simulink model "ai_neuron"  (R2020a)
settings: Solver=VariableStepAuto  StartTime=0.0  StopTime=30  RelTol=1e-3
libraries: xbsIndex_r4 x56, simulink x1
settings Model: Creator=Bunny1719  LastModifiedBy=asus

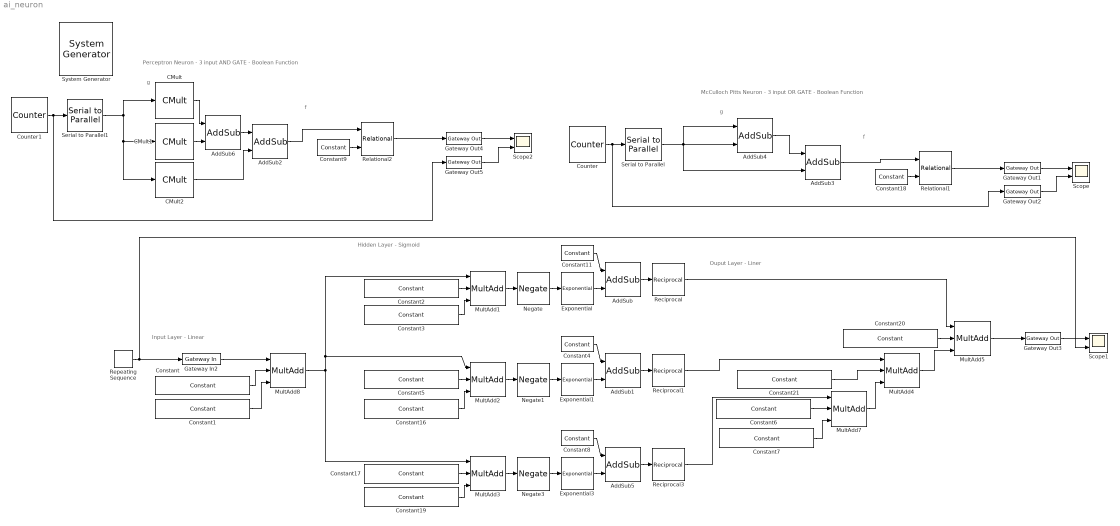
== system ai_neuron ==
  note: Ouput Layer - Liner
  note: Hidden Layer - Sigmoid
  note: Input Layer - Linear
  note: McCulloch Pitts Neuron - 3 input OR GATE - Boolean Function
  note: f
  note: g
  note: Perceptron Neuron - 3 input AND GATE - Boolean Function
  note: g
  note: f
  " System Generator" : xbsIndex_r4/ System Generator  Tag=genX  xilinxfamily=kintex7  part=xc7k325t  speed=-3  package=fbg676  synthesis_tool=Vivado  clock_wrapper=Clock Enables  directory=./netlist  proj_type=Vivado  Synth_file=Vivado Synthesis Defaults  Impl_file=Vivado Implementation Defaults  testbench=off  simulink_period=1  sysclk_period=10  dcm_input_clock_period=10  incr_netlist=off  trim_vbits=Everywhere in SubSystem  dbl_ovrd=According to Block Masks  core_generation=According to Block Masks  run_coregen=off  deprecated_control=off  eval_field=0  block_type=sysgen
  AddSub : xbsIndex_r4/AddSub  mode=Addition  use_carryin=off  use_carryout=off  en=off  latency=1  precision=Full  arith_type=Unsigned  n_bits=16  bin_pt=14  quantization=Truncate  overflow=Wrap  use_behavioral_HDL=off  hw_selection=Fabric  pipelined=off  dbl_ovrd=off  block_type=addsub
  AddSub1 : xbsIndex_r4/AddSub  mode=Addition  use_carryin=off  use_carryout=off  en=off  latency=1  precision=Full  arith_type=Unsigned  n_bits=16  bin_pt=14  quantization=Truncate  overflow=Wrap  use_behavioral_HDL=off  hw_selection=Fabric  pipelined=off  dbl_ovrd=off  block_type=addsub
  AddSub2 : xbsIndex_r4/AddSub  mode=Addition  use_carryin=off  use_carryout=off  en=off  latency=1  precision=User Defined  arith_type=Unsigned  n_bits=5  bin_pt=0  quantization=Truncate  overflow=Wrap  use_behavioral_HDL=off  hw_selection=Fabric  pipelined=off  dbl_ovrd=off  block_type=addsub
  AddSub3 : xbsIndex_r4/AddSub  mode=Addition  use_carryin=off  use_carryout=off  en=off  latency=1  precision=User Defined  arith_type=Unsigned  n_bits=3  bin_pt=0  quantization=Truncate  overflow=Wrap  use_behavioral_HDL=off  hw_selection=Fabric  pipelined=off  dbl_ovrd=off  block_type=addsub
  AddSub4 : xbsIndex_r4/AddSub  mode=Addition  use_carryin=off  use_carryout=off  en=off  latency=1  precision=User Defined  arith_type=Unsigned  n_bits=3  bin_pt=0  quantization=Truncate  overflow=Wrap  use_behavioral_HDL=off  hw_selection=Fabric  pipelined=off  dbl_ovrd=off  block_type=addsub
  AddSub5 : xbsIndex_r4/AddSub  mode=Addition  use_carryin=off  use_carryout=off  en=off  latency=1  precision=Full  arith_type=Unsigned  n_bits=16  bin_pt=14  quantization=Truncate  overflow=Wrap  use_behavioral_HDL=off  hw_selection=Fabric  pipelined=off  dbl_ovrd=off  block_type=addsub
  AddSub6 : xbsIndex_r4/AddSub  mode=Addition  use_carryin=off  use_carryout=off  en=off  latency=1  precision=User Defined  arith_type=Unsigned  n_bits=5  bin_pt=0  quantization=Truncate  overflow=Wrap  use_behavioral_HDL=off  hw_selection=Fabric  pipelined=off  dbl_ovrd=off  block_type=addsub
  CMult : xbsIndex_r4/CMult  const=1  gui_display_data_type=Fixed-point  const_n_bits=3  const_bin_pt=0  float_type=Single  exp_bits=8  fraction_bits=24  en=off  latency=1  precision=Full  arith_type="Signed  (2's comp)"  n_bits=16  bin_pt=14  quantization=Truncate  overflow=Wrap  use_behavioral_HDL=off  mem_type=Distributed RAM  pipeline=off  dbl_ovrd=off  block_type=cmult
  CMult1 : xbsIndex_r4/CMult  const=1  gui_display_data_type=Fixed-point  const_n_bits=3  const_bin_pt=0  float_type=Single  exp_bits=8  fraction_bits=24  en=off  latency=1  precision=Full  arith_type="Signed  (2's comp)"  n_bits=16  bin_pt=14  quantization=Truncate  overflow=Wrap  use_behavioral_HDL=off  mem_type=Distributed RAM  pipeline=off  dbl_ovrd=off  block_type=cmult
  CMult2 : xbsIndex_r4/CMult  const=1  gui_display_data_type=Fixed-point  const_n_bits=3  const_bin_pt=0  float_type=Single  exp_bits=8  fraction_bits=24  en=off  latency=2  precision=Full  arith_type="Signed  (2's comp)"  n_bits=16  bin_pt=14  quantization=Truncate  overflow=Wrap  use_behavioral_HDL=off  mem_type=Distributed RAM  pipeline=off  dbl_ovrd=off  block_type=cmult
  Constant : xbsIndex_r4/Constant  const=-0.6015088  gui_display_data_type=Floating-point  arith_type=Floating-point  n_bits=16  bin_pt=14  preci_type=Double  exp_width=8  frac_width=24  explicit_period=off  period=1  equ=P=C  opselect=C  inp2=PCIN>>17  opr=+  inp1=P  carry=CIN  dbl_ovrd=off  block_type=constant
  Constant1 : xbsIndex_r4/Constant  const=-3.04367  gui_display_data_type=Floating-point  arith_type=Floating-point  n_bits=16  bin_pt=14  preci_type=Double  exp_width=8  frac_width=24  explicit_period=off  period=1  equ=P=C  opselect=C  inp2=PCIN>>17  opr=+  inp1=P  carry=CIN  dbl_ovrd=off  block_type=constant
  Constant11 : xbsIndex_r4/Constant  const=1.0  gui_display_data_type=Floating-point  arith_type=Floating-point  n_bits=16  bin_pt=14  preci_type=Double  exp_width=8  frac_width=24  explicit_period=off  period=1  equ=P=C  opselect=C  inp2=PCIN>>17  opr=+  inp1=P  carry=CIN  dbl_ovrd=off  block_type=constant
  Constant16 : xbsIndex_r4/Constant  const=5.0102215  gui_display_data_type=Floating-point  arith_type=Floating-point  n_bits=16  bin_pt=14  preci_type=Double  exp_width=8  frac_width=24  explicit_period=off  period=1  equ=P=C  opselect=C  inp2=PCIN>>17  opr=+  inp1=P  carry=CIN  dbl_ovrd=off  block_type=constant
  Constant17 : xbsIndex_r4/Constant  const=0.7876907  gui_display_data_type=Floating-point  arith_type=Floating-point  n_bits=16  bin_pt=14  preci_type=Double  exp_width=8  frac_width=24  explicit_period=off  period=1  equ=P=C  opselect=C  inp2=PCIN>>17  opr=+  inp1=P  carry=CIN  dbl_ovrd=off  block_type=constant
  Constant18 : xbsIndex_r4/Constant  const=1  gui_display_data_type=Fixed-point  arith_type=Unsigned  n_bits=3  bin_pt=0  preci_type=Double  exp_width=8  frac_width=24  explicit_period=on  period=1  equ=P=C  opselect=C  inp2=PCIN>>17  opr=+  inp1=P  carry=CIN  dbl_ovrd=off  block_type=constant
  Constant19 : xbsIndex_r4/Constant  const=-1.3747003  gui_display_data_type=Floating-point  arith_type=Floating-point  n_bits=16  bin_pt=14  preci_type=Double  exp_width=8  frac_width=24  explicit_period=off  period=1  equ=P=C  opselect=C  inp2=PCIN>>17  opr=+  inp1=P  carry=CIN  dbl_ovrd=off  block_type=constant
  Constant2 : xbsIndex_r4/Constant  const=0.83689314  gui_display_data_type=Floating-point  arith_type=Floating-point  n_bits=16  bin_pt=14  preci_type=Double  exp_width=8  frac_width=24  explicit_period=off  period=1  equ=P=C  opselect=C  inp2=PCIN>>17  opr=+  inp1=P  carry=CIN  dbl_ovrd=off  block_type=constant
  Constant20 : xbsIndex_r4/Constant  const=-12.741189  gui_display_data_type=Floating-point  arith_type=Floating-point  n_bits=16  bin_pt=14  preci_type=Double  exp_width=8  frac_width=24  explicit_period=off  period=1  equ=P=C  opselect=C  inp2=PCIN>>17  opr=+  inp1=P  carry=CIN  dbl_ovrd=off  block_type=constant
  Constant21 : xbsIndex_r4/Constant  const=7.0409546  gui_display_data_type=Floating-point  arith_type=Floating-point  n_bits=16  bin_pt=14  preci_type=Double  exp_width=8  frac_width=24  explicit_period=off  period=1  equ=P=C  opselect=C  inp2=PCIN>>17  opr=+  inp1=P  carry=CIN  dbl_ovrd=off  block_type=constant
  Constant3 : xbsIndex_r4/Constant  const=6.2452445  gui_display_data_type=Floating-point  arith_type=Floating-point  n_bits=16  bin_pt=14  preci_type=Double  exp_width=8  frac_width=24  explicit_period=off  period=1  equ=P=C  opselect=C  inp2=PCIN>>17  opr=+  inp1=P  carry=CIN  dbl_ovrd=off  block_type=constant
  Constant4 : xbsIndex_r4/Constant  const=1.0  gui_display_data_type=Floating-point  arith_type=Floating-point  n_bits=16  bin_pt=14  preci_type=Double  exp_width=8  frac_width=24  explicit_period=off  period=1  equ=P=C  opselect=C  inp2=PCIN>>17  opr=+  inp1=P  carry=CIN  dbl_ovrd=off  block_type=constant
  Constant5 : xbsIndex_r4/Constant  const=-0.12644802  gui_display_data_type=Floating-point  arith_type=Floating-point  n_bits=16  bin_pt=14  preci_type=Double  exp_width=8  frac_width=24  explicit_period=off  period=1  equ=P=C  opselect=C  inp2=PCIN>>17  opr=+  inp1=P  carry=CIN  dbl_ovrd=off  block_type=constant
  Constant6 : xbsIndex_r4/Constant  const=14.252598  gui_display_data_type=Floating-point  arith_type=Floating-point  n_bits=16  bin_pt=14  preci_type=Double  exp_width=8  frac_width=24  explicit_period=off  period=1  equ=P=C  opselect=C  inp2=PCIN>>17  opr=+  inp1=P  carry=CIN  dbl_ovrd=off  block_type=constant
  Constant7 : xbsIndex_r4/Constant  const=5.2259626  gui_display_data_type=Floating-point  arith_type=Floating-point  n_bits=16  bin_pt=14  preci_type=Double  exp_width=8  frac_width=24  explicit_period=off  period=1  equ=P=C  opselect=C  inp2=PCIN>>17  opr=+  inp1=P  carry=CIN  dbl_ovrd=off  block_type=constant
  Constant8 : xbsIndex_r4/Constant  const=1.0  gui_display_data_type=Floating-point  arith_type=Floating-point  n_bits=16  bin_pt=14  preci_type=Double  exp_width=8  frac_width=24  explicit_period=off  period=1  equ=P=C  opselect=C  inp2=PCIN>>17  opr=+  inp1=P  carry=CIN  dbl_ovrd=off  block_type=constant
  Constant9 : xbsIndex_r4/Constant  const=21  gui_display_data_type=Fixed-point  arith_type=Unsigned  n_bits=5  bin_pt=0  preci_type=Double  exp_width=8  frac_width=24  explicit_period=on  period=1  equ=P=C  opselect=C  inp2=PCIN>>17  opr=+  inp1=P  carry=CIN  dbl_ovrd=off  block_type=constant
  Counter : xbsIndex_r4/Counter  cnt_type=Free Running  cnt_to=Inf  operation=Up  start_count=0  cnt_by_val=1  arith_type=Unsigned  n_bits=3  bin_pt=0  load_pin=off  rst=off  en=off  explicit_period=on  period=1  use_behavioral_HDL=off  implementation=Fabric  dbl_ovrd=off  block_type=counter
  Counter1 : xbsIndex_r4/Counter  cnt_type=Free Running  cnt_to=Inf  operation=Up  start_count=0  cnt_by_val=1  arith_type=Unsigned  n_bits=3  bin_pt=0  load_pin=off  rst=off  en=off  explicit_period=on  period=1  use_behavioral_HDL=off  implementation=Fabric  dbl_ovrd=off  block_type=counter
  Exponential : xbsIndex_r4/Exponential  flow_control=NonBlocking  axi_optimize_goal=Resources  bmg_use=NoUsage  latency=1  has_a_tlast=off  has_a_tuser=off  en=off  has_result_tready=off  has_underflow=off  has_overflow=off  fpo_op_type=exponential  rate=1  has_b_tlast=false  has_b_tuser=false  result_tlast_behv=1  has_divide_by_zero=false  has_invalid_op=false  block_type=exponential
      settings: infoedit=Blocking: Wait for data on all inputs, allow back-pressure.<br>NonBlocking: operate every cycle in which all inputs are valid, no back-pressure.
  Exponential1 : xbsIndex_r4/Exponential  flow_control=NonBlocking  axi_optimize_goal=Resources  bmg_use=NoUsage  latency=1  has_a_tlast=off  has_a_tuser=off  en=off  has_result_tready=off  has_underflow=off  has_overflow=off  fpo_op_type=exponential  rate=1  has_b_tlast=false  has_b_tuser=false  result_tlast_behv=1  has_divide_by_zero=false  has_invalid_op=false  block_type=exponential
      settings: infoedit=Blocking: Wait for data on all inputs, allow back-pressure.<br>NonBlocking: operate every cycle in which all inputs are valid, no back-pressure.
  Exponential3 : xbsIndex_r4/Exponential  flow_control=NonBlocking  axi_optimize_goal=Resources  bmg_use=NoUsage  latency=1  has_a_tlast=off  has_a_tuser=off  en=off  has_result_tready=off  has_underflow=off  has_overflow=off  fpo_op_type=exponential  rate=1  has_b_tlast=false  has_b_tuser=false  result_tlast_behv=1  has_divide_by_zero=false  has_invalid_op=false  block_type=exponential
      settings: infoedit=Blocking: Wait for data on all inputs, allow back-pressure.<br>NonBlocking: operate every cycle in which all inputs are valid, no back-pressure.
  Gateway In2 : xbsIndex_r4/Gateway In  gui_display_data_type=Floating-point  arith_type=Floating-point  n_bits=16  bin_pt=14  preci_type=Double  exp_width=8  frac_width=24  rows=1  columns=1  quantization="Round  (unbiased: +/- Inf)"  overflow=Saturate  period=1  UseAsADC=off  ADCChannel='1'  interface=None  automatic_assignment=on  address_offset=hex2dec('00')  intf_name=''  intf_description=''  default_value=0  timing_constraint=None  locs_specified=off  LOCs={}  io_standard={}  inherit_from_input=off  hdl_port=on  dbl_ovrd=off  block_type=gatewayin
  Gateway Out{1..2,4..5} (4 alike) : xbsIndex_r4/Gateway Out  inherit_from_input=off  hdl_port=on  rows=1  columns=1  UseAsDAC=off  DACChannel='1'  interface=None  automatic_assignment=on  address_offset=hex2dec('00')  intf_name=''  intf_description=''  timing_constraint=None  locs_specified=off  LOCs={}  io_standard={}  block_type=gatewayout
  Gateway Out3 : xbsIndex_r4/Gateway Out  inherit_from_input=on  hdl_port=on  rows=1  columns=1  UseAsDAC=off  DACChannel='1'  interface=None  automatic_assignment=on  address_offset=hex2dec('00')  intf_name=''  intf_description=''  timing_constraint=None  locs_specified=off  LOCs={}  io_standard={}  block_type=gatewayout
  MultAdd{1..5,7..8} (7 alike) : xbsIndex_r4/MultAdd  mode=Addition  en=off  infoeditControl=Fixed-point latency can be set to -1 or 0. The -1 selection will provide the optimum latency for max frequency for the given parameters.<br>Floating-point latency can be set to 0 or greater.  latency=0  precision=Full  arith_type=Unsigned  n_bits=16  bin_pt=14  block_type=multadd
  Negate : xbsIndex_r4/Negate  precision=Full  arith_type=Unsigned  n_bits=16  bin_pt=14  quantization=Truncate  overflow=Wrap  en=off  latency=1  dbl_ovrd=off  block_type=negate
  Negate1 : xbsIndex_r4/Negate  precision=Full  arith_type=Unsigned  n_bits=16  bin_pt=14  quantization=Truncate  overflow=Wrap  en=off  latency=1  dbl_ovrd=off  block_type=negate
  Negate3 : xbsIndex_r4/Negate  precision=Full  arith_type=Unsigned  n_bits=16  bin_pt=14  quantization=Truncate  overflow=Wrap  en=off  latency=1  dbl_ovrd=off  block_type=negate
  Reciprocal : xbsIndex_r4/Reciprocal  flow_control=NonBlocking  axi_optimize_goal=Resources  latency=1  has_a_tlast=off  has_a_tuser=off  en=off  has_result_tready=off  has_underflow=off  has_divide_by_zero=off  fpo_op_type=reciprocal  rate=1  has_b_tlast=false  has_b_tuser=false  result_tlast_behv=1  has_overflow=false  has_invalid_op=false  block_type=reciprocal
      settings: infoedit=Blocking: Wait for data on all inputs, allow back-pressure.<br>NonBlocking: operate every cycle in which all inputs are valid, no back-pressure.
  Reciprocal1 : xbsIndex_r4/Reciprocal  flow_control=NonBlocking  axi_optimize_goal=Resources  latency=1  has_a_tlast=off  has_a_tuser=off  en=off  has_result_tready=off  has_underflow=off  has_divide_by_zero=off  fpo_op_type=reciprocal  rate=1  has_b_tlast=false  has_b_tuser=false  result_tlast_behv=1  has_overflow=false  has_invalid_op=false  block_type=reciprocal
      settings: infoedit=Blocking: Wait for data on all inputs, allow back-pressure.<br>NonBlocking: operate every cycle in which all inputs are valid, no back-pressure.
  Reciprocal3 : xbsIndex_r4/Reciprocal  flow_control=NonBlocking  axi_optimize_goal=Resources  latency=1  has_a_tlast=off  has_a_tuser=off  en=off  has_result_tready=off  has_underflow=off  has_divide_by_zero=off  fpo_op_type=reciprocal  rate=1  has_b_tlast=false  has_b_tuser=false  result_tlast_behv=1  has_overflow=false  has_invalid_op=false  block_type=reciprocal
      settings: infoedit=Blocking: Wait for data on all inputs, allow back-pressure.<br>NonBlocking: operate every cycle in which all inputs are valid, no back-pressure.
  Relational1 : xbsIndex_r4/Relational  mode=a>=b  op_type=Bool  en=off  latency=1  dbl_ovrd=off  block_type=relational
  Relational2 : xbsIndex_r4/Relational  mode=a>=b  op_type=Bool  en=off  latency=1  dbl_ovrd=off  block_type=relational
  Repeating Sequence : simulink/Sources/Repeating Sequence  rep_seq_t=[0 35]  rep_seq_y=[-7 7]
  Scope : Scope  NumInputPorts=2
  Scope1 : Scope  NumInputPorts=2
  Scope2 : Scope  NumInputPorts=2
  Serial to Parallel : xbsIndex_r4/Serial to Parallel  input_order=Least Significant Word First  arith_type=Unsigned  output_bits=3  bin_pt=0  rst=off  en=off  latency=1  dbl_ovrd=off  block_type=s2p
      settings: infoedit=Groups of samples presented serially at the input become single samples presented at the output.
  Serial to Parallel1 : xbsIndex_r4/Serial to Parallel  input_order=Least Significant Word First  arith_type=Unsigned  output_bits=3  bin_pt=0  rst=off  en=off  latency=1  dbl_ovrd=off  block_type=s2p
      settings: infoedit=Groups of samples presented serially at the input become single samples presented at the output.
  wires:
  Constant2/1 -> MultAdd1/2
  Constant11/1 -> AddSub/1
  Exponential/1 -> AddSub/2
  Negate/1 -> Exponential/1
  MultAdd1/1 -> Negate/1
  AddSub/1 -> Reciprocal/1
  AddSub4/1 -> AddSub3/1
  Serial to Parallel/1 -> AddSub3/2, AddSub4/1, AddSub4/2
  AddSub3/1 -> Relational1/1
  Constant18/1 -> Relational1/2
  Relational1/1 -> Gateway Out1/1
  Counter/1 -> Gateway Out2/1, Serial to Parallel/1
  Gateway Out1/1 -> Scope/1
  Gateway Out2/1 -> Scope/2
  Gateway In2/1 -> MultAdd8/1
  MultAdd2/1 -> Negate1/1
  Negate1/1 -> Exponential1/1
  AddSub1/1 -> Reciprocal1/1
  Exponential1/1 -> AddSub1/2
  Constant4/1 -> AddSub1/1
  MultAdd3/1 -> Negate3/1
  Negate3/1 -> Exponential3/1
  AddSub5/1 -> Reciprocal3/1
  Exponential3/1 -> AddSub5/2
  Constant8/1 -> AddSub5/1
  MultAdd8/1 -> MultAdd1/1, MultAdd2/1, MultAdd3/1
  MultAdd7/1 -> MultAdd4/3
  Reciprocal3/1 -> MultAdd7/1
  Reciprocal1/1 -> MultAdd4/1
  MultAdd4/1 -> MultAdd5/3
  Reciprocal/1 -> MultAdd5/1
  MultAdd5/1 -> Gateway Out3/1
  Gateway Out3/1 -> Scope1/1
  Repeating Sequence/1 -> Gateway In2/1, Scope1/2
  Constant/1 -> MultAdd8/2
  Constant1/1 -> MultAdd8/3
  Constant3/1 -> MultAdd1/3
  Constant5/1 -> MultAdd2/2
  Constant17/1 -> MultAdd3/2
  Constant19/1 -> MultAdd3/3
  Constant16/1 -> MultAdd2/3
  Constant20/1 -> MultAdd5/2
  Constant21/1 -> MultAdd4/2
  Constant6/1 -> MultAdd7/2
  Constant7/1 -> MultAdd7/3
  Gateway Out5/1 -> Scope2/2
  Relational2/1 -> Gateway Out4/1
  AddSub2/1 -> Relational2/1
  Counter1/1 -> Gateway Out5/1, Serial to Parallel1/1
  Constant9/1 -> Relational2/2
  Gateway Out4/1 -> Scope2/1
  CMult/1 -> AddSub6/1
  AddSub6/1 -> AddSub2/1
  CMult1/1 -> AddSub6/2
  CMult2/1 -> AddSub2/2
  Serial to Parallel1/1 -> CMult/1, CMult1/1, CMult2/1
